simulink model "demo1"  (R2022a)
settings: Solver=VariableStepAuto  StartTime=0.0  StopTime=10  RelTol=1e-3
libraries: spsDiodeLib x6, spsPVArrayLib x6, spsVoltageMeasurementLib x3, spsCurrentMeasurementLib x1, spsIdealSwitchLib x1, spsSeriesRLCBranchLib x1, spspowerguiLib x1
settings Model: Creator=Dell  LastModifiedBy=Dell

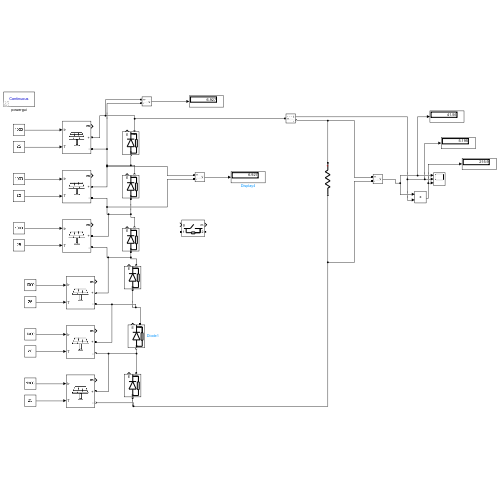
[thumbnail: Simulink's stored preview of the top-level diagram]
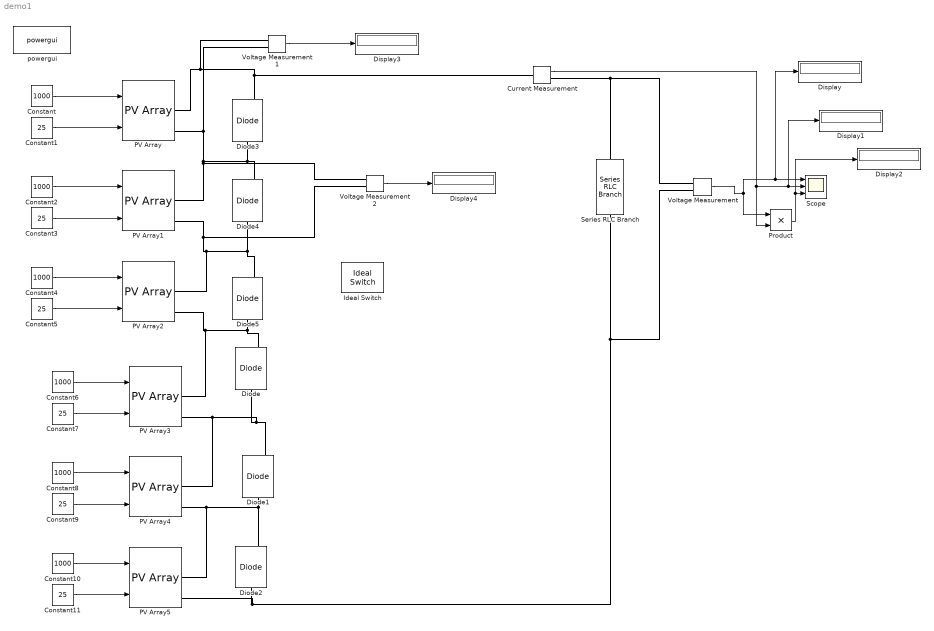
== system demo1 ==
  Constant{,2,4,6,8,10} (6 alike) : Constant  Value=1000
  Constant{1,3,5,7,9,11} (6 alike) : Constant  Value=25
  Current Measurement : spsCurrentMeasurementLib/Current Measurement  PhasorSimulation=off  OutputType=Complex  PSBequivalent=0
  Diode{,1..5} (6 alike) : spsDiodeLib/Diode  Ron=0.001  Lon=0  Vf=0.8  IC=0  UseSnubber=0  Rs=500  Cs=250e-9  Measurements=on
  Display{,1..4} (5 alike) : Display
  Ideal Switch : spsIdealSwitchLib/Ideal Switch  Ron=0.001  Lon=0  IC=0  Rs=1e5  Cs=inf  Measurements=on
  PV Array{,1..5} (6 alike) : spsPVArrayLib/PV Array  Npar=1  Nser=1  PlotType=array @ 1000 W/m2 & specified temperatures  S_vec="[ 1000  500  100 ]"  Temp_C_vec="[ 45 25  ]"  ModuleName=Aavid Solar ASMS-165P  PlotWhenSelected=off  Pm=164.85  Ncell=72  Voc=43.5  Isc=5.25  Vm=35  Im=4.71  beta_Voc_pc=-0.393  alpha_Isc_pc=0.03  beta_Voc=-0.17095  alpha_Isc=0.001575  IL=5.2764  I0=4.9875e-10  nI=1.0218  Rsh=125.0069  Rs=0.62818  RobustModel=off  RobustCellTemperature=313.3991  BAL=on  Tc=1e-6  Tfilter=5e-5
  Product : Product
  Scope : Scope  NumInputPorts=3
  Series RLC Branch : spsSeriesRLCBranchLib/Series RLC Branch  LConnTagsString=__new0  RConnTagsString=__new0  BranchType=R  Resistance=8  Inductance=1e-3  SetiL0=off  InitialCurrent=0  Capacitance=1e-6  Setx0=off  InitialVoltage=0  Measurements=None
  Voltage Measurement : spsVoltageMeasurementLib/Voltage Measurement  PhasorSimulation=off  OutputType=Complex  PSBequivalent=0
  Voltage Measurement1 : spsVoltageMeasurementLib/Voltage Measurement  PhasorSimulation=off  OutputType=Complex  PSBequivalent=0
  Voltage Measurement2 : spsVoltageMeasurementLib/Voltage Measurement  PhasorSimulation=off  OutputType=Complex  PSBequivalent=0
  powergui : spspowerguiLib/powergui  Priority=1  SimulationMode=Continuous  SampleTime=50e-6  frequency=60  Iterations=50  frequencyindice=0  Pbase=100e6  ErrMax=1e-4  UnitsV=kV  UnitsW=MW  buscounter=0  FunctionMessages=off  echomessages=off  EnableUseOfTLC=off  CurrentSourceSwitches=off  DisableSnubberDevices=off  DisableRonSwitches=off  DisableVfSwitches=off  DisplayEquations=off  AutomaticDiscreteSolvers=off  SolverType=Tustin/Backward Euler (TBE)  Interpol=off  ExternalGateDelay=off  methode=off  Ts=100  x0status=blocks  SPID=on  SwTol=0  HookPort=off  NonlinearTolerance=1e-4  nMaxIteration=100  ContinueOnMaxIteration=off  RestoreLinks=warning  ResistiveCurrentMeasurement=off  Frange=[0:2:500]  Ylog=off  Xlog=on  ShowGrid=off  save=off  variable=ZData  structure=0  ZoomFFT=off  StartTime=0.0  cycles=1  DisplayStyle=1  fundamental=60  FreqAxis=off  MaxFrequency=1000  frequencyindicesteady=1  RmsSteady=1  display=off
  wires:
  Constant/1 -> PV Array/1
  Constant1/1 -> PV Array/2
  Constant2/1 -> PV Array1/1
  Constant3/1 -> PV Array1/2
  Constant4/1 -> PV Array2/1
  Constant5/1 -> PV Array2/2
  Voltage Measurement/1 -> Display/1, Scope/1, Product/1
  Current Measurement/1 -> Product/2, Display1/1, Scope/2
  Product/1 -> Display2/1, Scope/3
  Constant6/1 -> PV Array3/1
  Constant7/1 -> PV Array3/2
  Constant8/1 -> PV Array4/1
  Constant9/1 -> PV Array4/2
  Constant10/1 -> PV Array5/1
  Constant11/1 -> PV Array5/2
  Voltage Measurement1/1 -> Display3/1
  Voltage Measurement2/1 -> Display4/1
  connections:
  Diode1/LConn1 -- PV Array5/RConn1 -- PV Array4/RConn2 -- Diode2/RConn1
  Diode/LConn1 -- PV Array4/RConn1 -- PV Array3/RConn2 -- Diode1/RConn1
  Voltage Measurement/LConn2 -- Series RLC Branch/RConn1 -- PV Array5/RConn2 -- Diode2/LConn1
  Voltage Measurement/LConn1 -- Series RLC Branch/LConn1 -- Current Measurement/RConn1
  Diode3/LConn1 -- PV Array1/RConn1 -- Voltage Measurement2/LConn1 -- Voltage Measurement1/LConn2 -- PV Array/RConn2 -- Diode4/RConn1
  Diode4/LConn1 -- Voltage Measurement2/LConn2 -- PV Array1/RConn2 -- PV Array2/RConn1 -- Diode5/RConn1
  Diode/RConn1 -- PV Array3/RConn1 -- PV Array2/RConn2 -- Diode5/LConn1
  PV Array/RConn1 -- Voltage Measurement1/LConn1 -- Current Measurement/LConn1 -- Diode3/RConn1
